simulink model "FBL_Plant"  (R2024b)
settings: Solver=ode45  StartTime=0.0  StopTime=300  MaxStep=0.5  RelTol=1e-5
settings Model: Creator=Denilson Nicolau  LastModifiedBy=dd364
settings DebuggingCC: UnconnectedInputMsg=warning  UnconnectedOutputMsg=warning  UnconnectedLineMsg=warning
settings ModelReferenceCC: EnableRefExpFcnMdlSchedulingChecks=on
settings RTWCC: GPUComputeCapability=3.5  DLArmComputeVersion=19.05

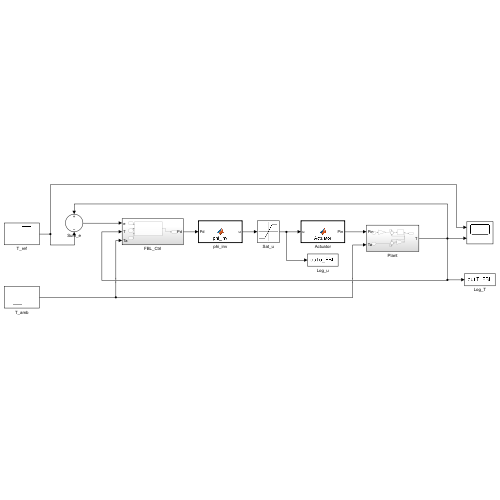
[thumbnail: Simulink's stored preview of the top-level diagram]
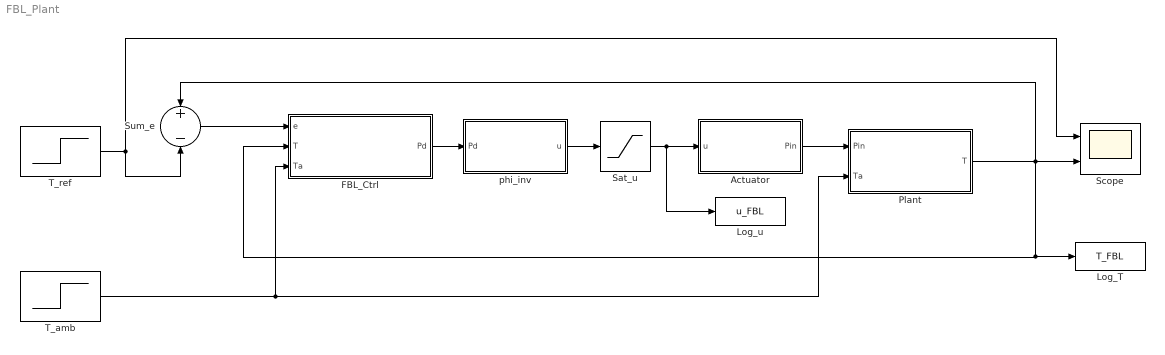
== system FBL_Plant ==
  Actuator : MATLAB Function  TreatAsAtomicUnit=on
  FBL_Ctrl : Subsystem
  Log_T : ToWorkspace  VariableName=T_FBL  SaveFormat=Timeseries  SampleTime=-1
  Log_u : ToWorkspace  VariableName=u_FBL  SaveFormat=Timeseries  SampleTime=-1
  Plant : Subsystem
  Sat_u : Saturate  UpperLimit=1.2  LowerLimit=0
  Scope : Scope  NumInputPorts=2
  Sum_e : Sum  Inputs=+-
  T_amb : Step  Time=150  Before=25  After=30  SampleTime=0
  T_ref : Step  Time=0  Before=25  After=70  SampleTime=0
  phi_inv : MATLAB Function  TreatAsAtomicUnit=on
  wires:
  Plant/1(T) -> Scope/2, FBL_Ctrl/2(T), Log_T/1, Sum_e/1
  T_ref/1 -> Sum_e/2, Scope/1
  Sum_e/1 -> FBL_Ctrl/1(e)
  T_amb/1 -> FBL_Ctrl/3(Ta), Plant/2(Ta)
  FBL_Ctrl/1(Pd) -> phi_inv/1(Pd)
  phi_inv/1(u) -> Sat_u/1
  Sat_u/1 -> Log_u/1, Actuator/1(u)
  Actuator/1(Pin) -> Plant/1(Pin)

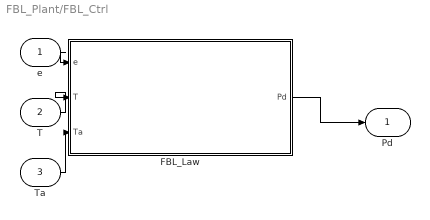
== system FBL_Plant/FBL_Ctrl ==
  e : Inport
  T : Inport  Port=2
  Ta : Inport  Port=3
  FBL_Law : MATLAB Function  TreatAsAtomicUnit=on
  Pd : Outport
  wires:
  e/1 -> FBL_Law/1(e)
  T/1 -> FBL_Law/2(T)
  Ta/1 -> FBL_Law/3(Ta)
  FBL_Law/1(Pd) -> Pd/1

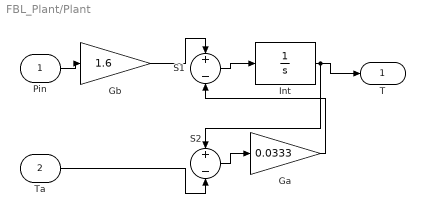
== system FBL_Plant/Plant ==
  Pin : Inport
  Ta : Inport  Port=2
  Ga : Gain  Gain=0.0333
  Gb : Gain  Gain=1.6
  Int : Integrator  InitialCondition=25
  S1 : Sum  Inputs=+-
  S2 : Sum  Inputs=+-
  T : Outport
  wires:
  Pin/1 -> Gb/1
  Gb/1 -> S1/1
  Ga/1 -> S1/2
  S1/1 -> Int/1
  Int/1 -> T/1, S2/1
  Ta/1 -> S2/2
  S2/1 -> Ga/1

== matlab function FBL_Plant/phi_inv ==
  data: Pd input; u output
function u = phi_inv(Pd)
%%#codegen
  Pd = max(1e-6, min(2.42, double(Pd)));
  u  = (log10(200*Pd) + 1) / 4;
end

== matlab function FBL_Plant/FBL_Ctrl/FBL_Law ==
  data: e input; Pd output; T input; Ta input
function Pd = FBL_Law(e, T, Ta)
  alpha = 0.0333;
  beta  = 1.6;
  k1    = 1.5;
  Pd    = (1/beta)*(alpha*(double(T)-double(Ta))-k1*double(e));
  Pd    = max(0, min(2.42, Pd));
end

== matlab function FBL_Plant/Actuator ==
  data: u input; Pin output
function Pin = Actuator(u)
%%#codegen
  Pin = (10^(4*double(u) - 1)) / 200;
end
